simulink model "CIC_HDL_Coder"  (R2024a)
settings: Solver=VariableStepDiscrete  StartTime=0.0  StopTime=10.0  MaxStep=1/1000000  RelTol=1e-3
libraries: hdlsllib x1
settings Model: Creator=Aleksandr  LastModifiedBy=Aleksandr
settings OptimizationCC: BlockReduction=off  ConditionallyExecuteInputs=off
settings DebuggingCC: SingleTaskRateTransMsg=error

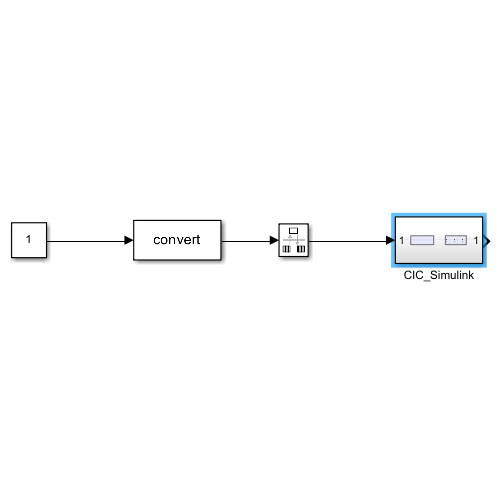
[thumbnail: Simulink's stored preview of the top-level diagram]
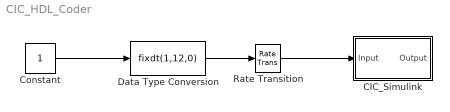
== system CIC_HDL_Coder ==
  CIC_Simulink : Subsystem  Tag=FilterWizardSubSystem
      settings: ErrorFcn=dspFilterRealizedInBasicElemsAlgLoopErrFcnCallback
  Constant : Constant  OutDataTypeStr=fixdt(1,12,0)  SampleTime=1/1000000
  Data Type Conversion : DataTypeConversion  OutDataTypeStr=fixdt(1,12,0)  SaturateOnIntegerOverflow=off  RndMeth=Floor
  Rate Transition : RateTransition  OutPortSampleTime=1/1000000
  wires:
  Rate Transition/1 -> CIC_Simulink/1(Input)
  Data Type Conversion/1 -> Rate Transition/1
  Constant/1 -> Data Type Conversion/1

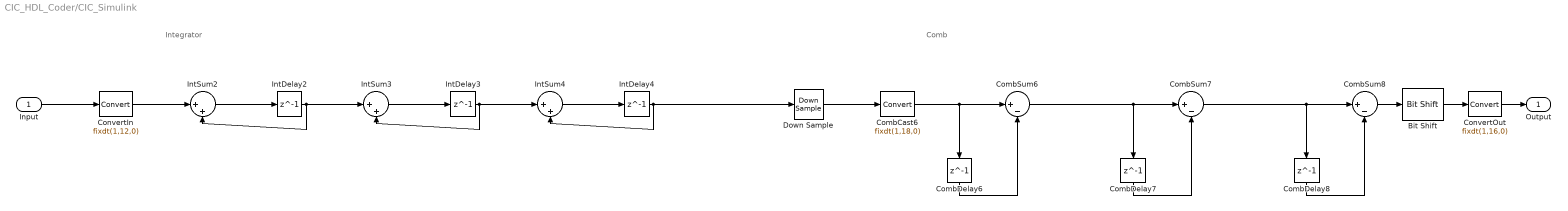
== system CIC_HDL_Coder/CIC_Simulink ==
  note: Comb
  note: Integrator
  Input : Inport
  Bit Shift : hdlsllib/Logic and Bit Operations/Bit Shift  mode=Shift Right Logical  N=2
  CombCast6 : DataTypeConversion  OutDataTypeStr=fixdt(1,18,0)  SaturateOnIntegerOverflow=off  RndMeth=Floor
  CombDelay6 : Delay  DelayLength=1  InitialCondition=0
  CombDelay7 : Delay  DelayLength=1  InitialCondition=0
  CombDelay8 : Delay  DelayLength=1  InitialCondition=0
  CombSum6 : Sum  Inputs=|+-  OutDataTypeStr=fixdt(1,18,0)  AccumDataTypeStr=fixdt(1,18,0)
  CombSum7 : Sum  Inputs=|+-  OutDataTypeStr=fixdt(1,18,0)  AccumDataTypeStr=fixdt(1,18,0)
  CombSum8 : Sum  Inputs=|+-  OutDataTypeStr=fixdt(1,18,0)  AccumDataTypeStr=fixdt(1,18,0)
  ConvertIn : DataTypeConversion  OutDataTypeStr=fixdt(1,12,0)  RndMeth=Nearest
  ConvertOut : DataTypeConversion  OutDataTypeStr=fixdt(1,16,0)  SaturateOnIntegerOverflow=off  RndMeth=Floor
  Down Sample : DownSample  N=4  RateOptions=Allow multirate processing  AllowArbitraryFixedInput=on
  IntDelay2 : Delay  DelayLength=1  InitialCondition=0
  IntDelay3 : Delay  DelayLength=1  InitialCondition=0
  IntDelay4 : Delay  DelayLength=1  InitialCondition=0
  IntSum2 : Sum  Inputs=|++  OutDataTypeStr=fixdt(1,18,0)  AccumDataTypeStr=fixdt(1,18,0)
  IntSum3 : Sum  Inputs=|++  OutDataTypeStr=fixdt(1,18,0)  AccumDataTypeStr=fixdt(1,18,0)
  IntSum4 : Sum  Inputs=|++  OutDataTypeStr=fixdt(1,18,0)  AccumDataTypeStr=fixdt(1,18,0)
  Output : Outport
  wires:
  Input/1 -> ConvertIn/1
  ConvertIn/1 -> IntSum2/1
  IntSum2/1 -> IntDelay2/1
  IntDelay2/1 -> IntSum2/2, IntSum3/1
  IntSum3/1 -> IntDelay3/1
  IntDelay3/1 -> IntSum3/2, IntSum4/1
  IntSum4/1 -> IntDelay4/1
  IntDelay4/1 -> IntSum4/2, Down Sample/1
  Down Sample/1 -> CombCast6/1
  CombSum6/1 -> CombSum7/1, CombDelay7/1
  CombDelay6/1 -> CombSum6/2
  CombCast6/1 -> CombSum6/1, CombDelay6/1
  CombSum7/1 -> CombSum8/1, CombDelay8/1
  CombDelay7/1 -> CombSum7/2
  CombSum8/1 -> Bit Shift/1
  CombDelay8/1 -> CombSum8/2
  ConvertOut/1 -> Output/1
  Bit Shift/1 -> ConvertOut/1
